simulink model "system11"  (Simulink 4.00)
settings: Solver=ode45  StartTime=0.0  StopTime=10.0  RelTol=1e-3
libraries: simulink_extras x4, cstblocks x2
settings Model: LastModifiedBy=Administrator  BlockReductionOpt=off

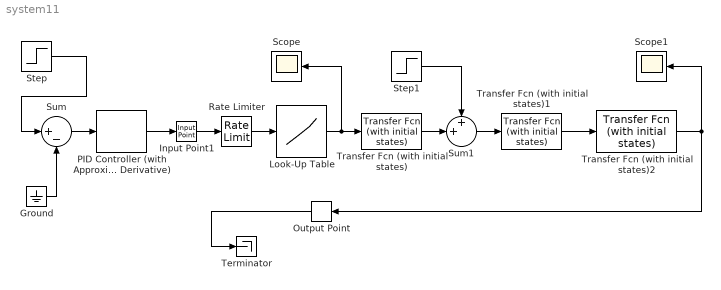
== system system11 ==
  Ground : Ground
  Input Point1 : cstblocks/Input Point
  Look-Up Table : Lookup  InputValues=[-50. -15,- 10, 0, 10, 15, 50]  OutputValues=[-15, -12, -10, 0, 10, 12, 15]
  Output Point : cstblocks/Output Point  Orientation=left
  PID Controller (with Approximate Derivative) : simulink_extras/Additional Linear/PID Controller (with Approximate Derivative)  P=10  I=8  D=1  N=20
  Rate Limiter : RateLimiter  RisingSlewLimit=50  FallingSlewLimit=-50
  Scope : Scope
      settings: TimeRange=auto  YMin=-5  YMax=5  SaveToWorkspace=off  SaveName=ScopeData  LimitDataPoints=on  MaxDataPoints=5000
  Scope1 : Scope
      settings: TimeRange=auto  YMin=-5  YMax=5  SaveToWorkspace=off  LimitDataPoints=on  MaxDataPoints=5000
  Step : Step  Time=0  Before=0  After=1  SampleTime=0
  Step1 : Step  Time=0  Before=0  After=0  SampleTime=0
  Sum : Sum  Inputs=|+-  SaturateOnIntegerOverflow=on
  Sum1 : Sum  Inputs=++|  SaturateOnIntegerOverflow=on
  Terminator : Terminator
  Transfer Fcn (with initial states) : simulink_extras/Additional Linear/Transfer Fcn (with initial states)  N=[1]  D="[1  1]"  X0=0
  Transfer Fcn (with initial states)1 : simulink_extras/Additional Linear/Transfer Fcn (with initial states)  N=[1]  D="[1  1]"  X0=0
  Transfer Fcn (with initial states)2 : simulink_extras/Additional Linear/Transfer Fcn (with initial states)  N=[1]  D=[1 2 8]  X0=0
  wires:
  Sum/1 -> PID Controller (with Approximate Derivative)/1
  Transfer Fcn (with initial states)/1 -> Sum1/2
  Step1/1 -> Sum1/1
  PID Controller (with Approximate Derivative)/1 -> Input Point1/1
  Sum1/1 -> Transfer Fcn (with initial states)1/1
  Transfer Fcn (with initial states)2/1 -> Output Point/1, Scope1/1
  Transfer Fcn (with initial states)1/1 -> Transfer Fcn (with initial states)2/1
  Rate Limiter/1 -> Look-Up Table/1
  Look-Up Table/1 -> Transfer Fcn (with initial states)/1, Scope/1
  Ground/1 -> Sum/2
  Output Point/1 -> Terminator/1
  Input Point1/1 -> Rate Limiter/1
  Step/1 -> Sum/1
